simulink model "Single_current_Vin_Iout_integrator_method"  (R2024a)
settings: Solver=VariableStepAuto  StartTime=0.0  StopTime=10.0  RelTol=1e-3
values from neighbouring files (symbols this model uses):
  C = 10    [Single_current_Vin_Vc_Iout_parameters.mat]
  L = 20    [Single_current_Vin_Vc_Iout_parameters.mat]
  R = 5    [Single_current_Vin_Vc_Iout_parameters.mat]
settings Model: Creator=nassa  LastModifiedBy=nassa

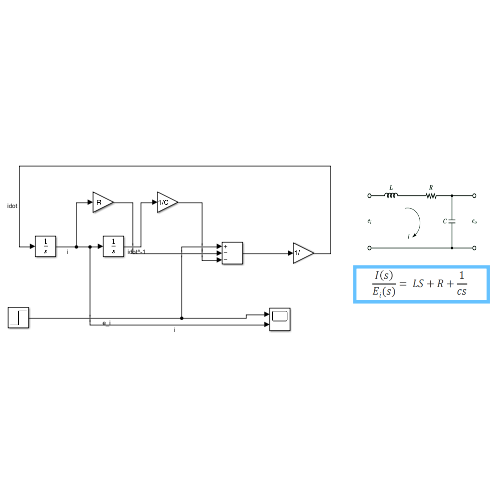
[thumbnail: Simulink's stored preview of the top-level diagram]
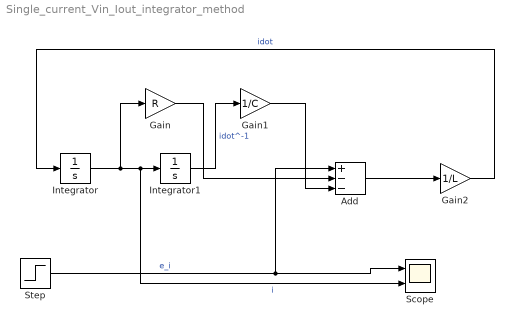
== system Single_current_Vin_Iout_integrator_method ==
  Add : Sum  Inputs=+--
  Gain : Gain  Gain=R
  Gain1 : Gain  Gain=1/C
  Gain2 : Gain  Gain=1/L
  Integrator : Integrator
  Integrator1 : Integrator
  Scope : Scope  NumInputPorts=2
  Step : Step  SampleTime=0
  wires:
  Integrator1/1 -> Gain1/1  "idot^-1"
  Integrator/1 -> Gain/1, Scope/2, Integrator1/1  "i"
  Gain2/1 -> Integrator/1  "idot"
  Gain/1 -> Add/2
  Gain1/1 -> Add/3
  Add/1 -> Gain2/1
  Step/1 -> Scope/1, Add/1  "e_i"
